simulink model "A3"  (R2026a)
settings: Solver=VariableStepAuto  StopTime=0.5
settings Model: Creator=Mandisa Dlamini  LastModifiedBy=Mandisa Dlamini

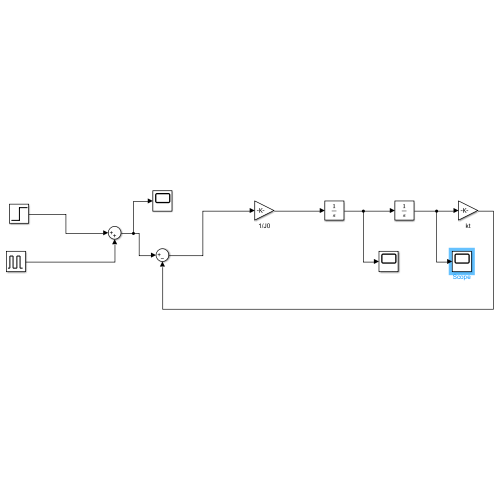
[thumbnail: Simulink's stored preview of the top-level diagram]
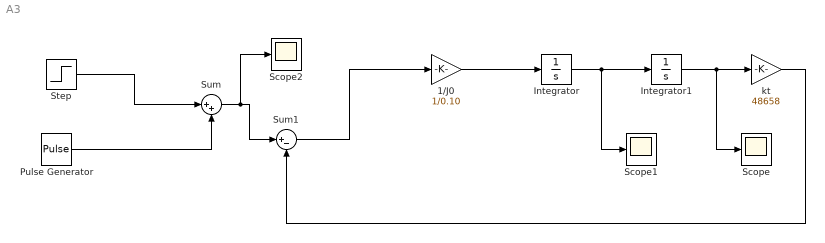
== system A3 ==
  1/J0 : Gain  Gain=1/0.10
  Integrator : Integrator
  Integrator1 : Integrator
  Pulse Generator : DiscretePulseGenerator  PulseType=Time based  Amplitude=-1000  Period=0.06  PulseWidth=6.25
  Scope : Scope
      settings: ActiveDisplayYMinimum=-0.028303452856664926  ActiveDisplayYMaximum=0.06948739117937644
  Scope1 : Scope
      settings: ActiveDisplayYMinimum=-34.124438852563443  ActiveDisplayYMaximum=34.138864306954424
  Scope2 : Scope
      settings: ActiveDisplayYMinimum=-1  ActiveDisplayYMaximum=1  DataLoggingVariableName=ScopeData2
  Step : Step  Time=0  FinalValue=1000  SampleTime=0
  Sum : Sum  Inputs=|++
  Sum1 : Sum  Inputs=|+-
  kt : Gain  Gain=48658
  wires:
  Step/1 -> Sum/1
  Pulse Generator/1 -> Sum/2
  Sum/1 -> Scope2/1, Sum1/1
  Sum1/1 -> 1/J0/1
  1/J0/1 -> Integrator/1
  Integrator/1 -> Scope1/1, Integrator1/1
  Integrator1/1 -> Scope/1, kt/1
  kt/1 -> Sum1/2
